simulink model "masa_resorte_amortiguador"  (R2024a)
settings: Solver=VariableStepAuto  StartTime=0.0  StopTime=10.0  RelTol=1e-3
model workspace (MAT data in the model file):
  k1 = 1
  k2 = 1
  m = 1

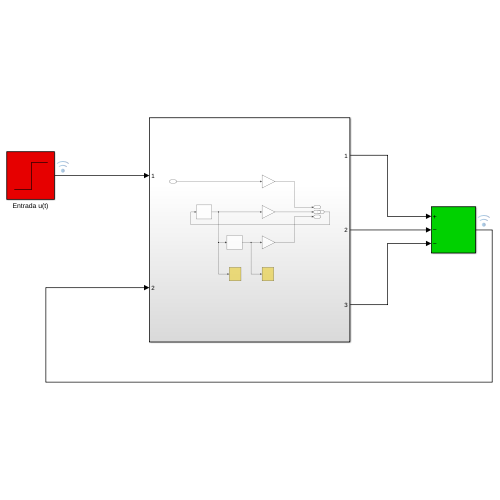
[thumbnail: Simulink's stored preview of the top-level diagram]
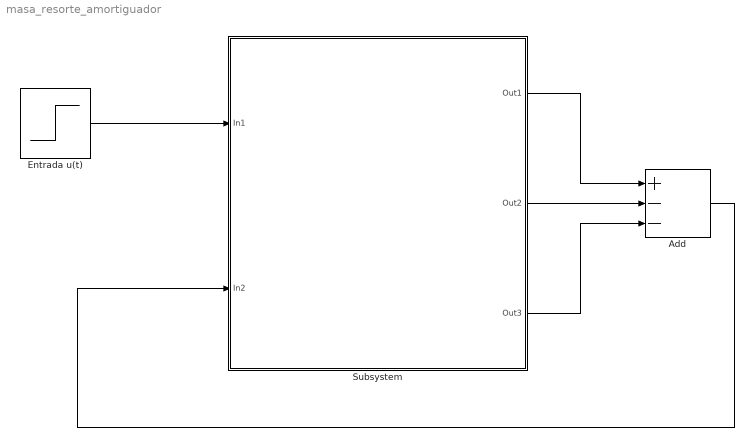
== system masa_resorte_amortiguador ==
  Add : Sum  Inputs=+--
  Entrada u(t) : Step  Time=2  After=10  SampleTime=0
  Subsystem : Subsystem
  wires:
  Entrada u(t)/1 -> Subsystem/1(In1)
  Add/1 -> Subsystem/2(In2)
  Subsystem/1(Out1) -> Add/1
  Subsystem/2(Out2) -> Add/2
  Subsystem/3(Out3) -> Add/3

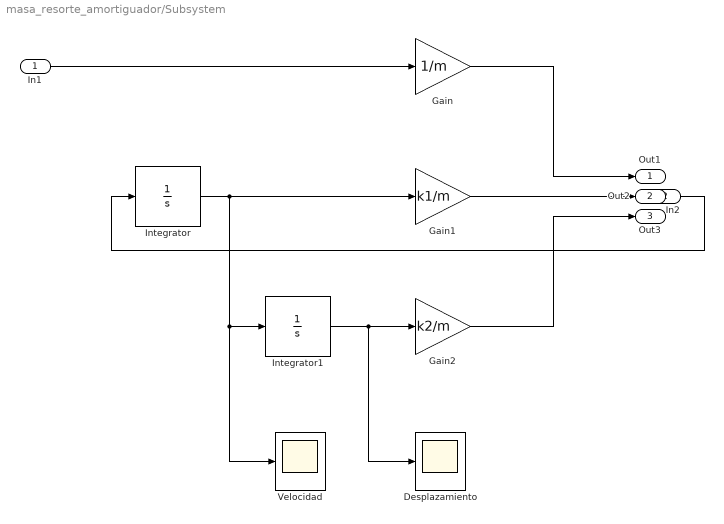
== system masa_resorte_amortiguador/Subsystem ==
  In1 : Inport
  In2 : Inport  Port=2
  Desplazamiento : Scope
  Gain : Gain  Gain=1/m
  Gain1 : Gain  Gain=k1/m
  Gain2 : Gain  Gain=k2/m
  Integrator : Integrator
  Integrator1 : Integrator
  Velocidad : Scope
  Out1 : Outport
  Out2 : Outport  Port=2
  Out3 : Outport  Port=3
  wires:
  In2/1 -> Integrator/1
  Integrator1/1 -> Desplazamiento/1, Gain2/1
  Integrator/1 -> Velocidad/1, Integrator1/1, Gain1/1
  In1/1 -> Gain/1
  Gain1/1 -> Out2/1
  Gain2/1 -> Out3/1
  Gain/1 -> Out1/1
